simulink model "DAQ"  (R2024a)
settings: Solver=VariableStepAuto  StartTime=0.0  StopTime=inf  RelTol=1e-3
undefined symbols (not defined in the file): daq
libraries: instrumentseriallib x2, daqlib x1
settings Model: Creator=JayHP  LastModifiedBy=JayHP

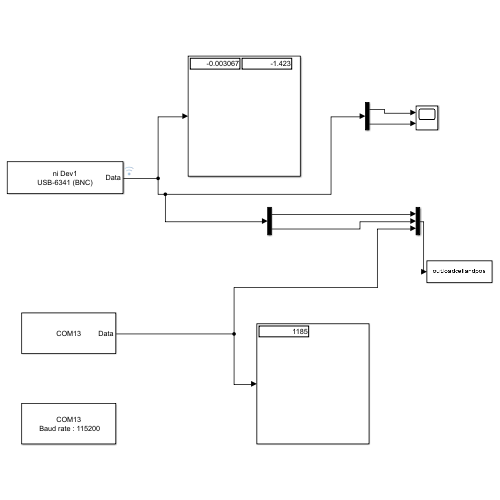
[thumbnail: Simulink's stored preview of the top-level diagram]
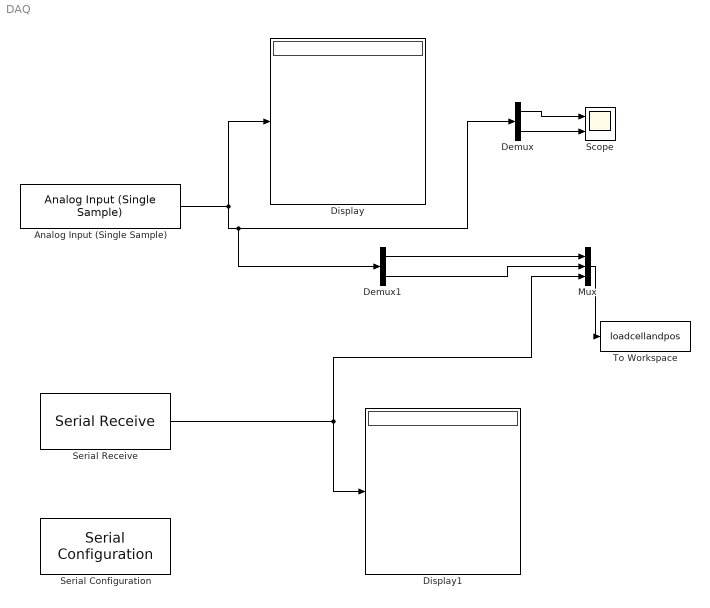
== system DAQ ==
  Analog Input (Single Sample) : daqlib/Analog Input (Single Sample)  DeviceMenu=ni Dev1 (USB-6341 (BNC))  Device=ni Dev1 (USB-6341 (BNC))  ObjConstructor=daq.createSession('ni')  BlockSampleTime=0.001  NChannelsSelected=2  Channels=1$ai0$$Dev1$1$4$3$1$#1$ai1$$Dev1$1$4$3$1$#0$ai2$$Dev1$1$4$3$1$#0$ai3$$Dev1$1$4$3$1$#0$ai4$$Dev1$1$4$3$1$#0$ai5$$Dev1$1$4$3$1$#0$ai6$$Dev1$1$4$3$1$#0$ai7$$Dev1$1$4$3$1$#0$ai8$$Dev1$1$4$1$1$#0$ai9$$Dev1$1$4$1$1$#0$ai10$$Dev1$1$4$1$1$#0$ai11$$Dev1$1$4$1$1$#0$ai12$$Dev1$1$4$1$1$#0$ai13$$Dev1$1$4$1$1$#0$ai14$$Dev1$1$4$1$1$#0$ai15$$Dev1$1$4$1$1$#  NPorts=1 for all channels  OutputTimestamp=off
  Demux : Demux  Outputs=2
  Demux1 : Demux  Outputs=2
  Display : Display
  Display1 : Display
  Mux : Mux  Inputs=3
  Scope : Scope  NumInputPorts=2
  Serial Configuration : instrumentseriallib/Serial Configuration  Priority=-200000  PortSel=COM13  Port=COM13  ComPort=COM13  BaudRate=115200  DataBits=8  Parity=none  StopBits=1  ByteOrder=little-endian  FlowControl=none  Timeout=10  SimulateUsing=Interpreted execution  BlockInModel=on  aMode=1
  Serial Receive : instrumentseriallib/Serial Receive  Priority=1  PortSel=COM13  Port=COM13  ComPort=COM13  DataType=double  SaveDataType=uint8  ToggleHeader=off  Header=[]  ToggleDataSize=on  DataSize=[1 1]  ToggleTerminator=off  Terminator=<none>  CustomTerminator=[]  InputFormat=Column major  EnableBlockingMode=on  ActionDataUnavailable=Output last received value  ActionWhenDataUnavailable=Output last received value  CustomValue=0  SampleTime=0.001  SimulateUsing=Interpreted execution  BlockInModel=on  aMode=1
  To Workspace : ToWorkspace  VariableName=loadcellandpos  SaveFormat=Timeseries  SampleTime=-1
  wires:
  Analog Input (Single Sample)/1 -> Demux1/1, Demux/1, Display/1
  Demux/1 -> Scope/1
  Demux/2 -> Scope/2
  Serial Receive/1 -> Mux/3, Display1/1
  Demux1/1 -> Mux/1
  Demux1/2 -> Mux/2
  Mux/1 -> To Workspace/1
